simulink model "mtuner_process"  (Simulink 3.00)
libraries: mathlib x4, analoglib x3, genlib x2, execlib x1, modellib x1

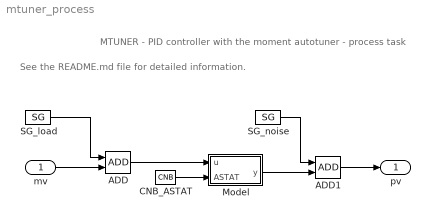
== system mtuner_process ==
  note: See the README.md file for detailed information.
  note: MTUNER - PID controller with the moment autotuner - process task
  mv : Inport  Port=1
  ADD : mathlib/ADD
  ADD1 : mathlib/ADD
  CNB_ASTAT : mathlib/CNB  YCN=off
  Model : Subsystem
      mask Type: REX sequence
  SG_load : genlib/SG  isig=1: SINE  amp=0  freq=0.01  phase=0  ifrunit=1: Hz  iphunit=1: DEGREE  offset=0
  SG_noise : genlib/SG  isig=4: RANDOM  amp=0  freq=0.01  phase=0  ifrunit=1: Hz  iphunit=1: DEGREE  offset=0
  pv : Outport  Port=1
  wires:
  ADD/1 -> Model/1(u)
  ADD1/1 -> pv/1
  CNB_ASTAT/1 -> Model/2(ASTAT)
  Model/1(y) -> ADD1/2
  SG_load/1 -> ADD/1
  SG_noise/1 -> ADD1/1
  mv/1 -> ADD/2

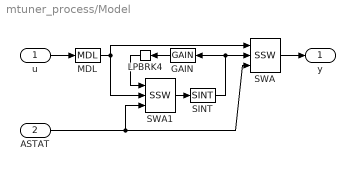
== system mtuner_process/Model ==
  u : Inport  Port=1
  ASTAT : Inport  Port=2
  GAIN : mathlib/GAIN  Orientation=left  k=-1
  LPBRK4 : execlib/LPBRK  Orientation=left
  MDL : modellib/MDL  k0=1  del=0  tau1=10  tau2=2  nmax=100
  SINT : analoglib/SINT  ti=1  y0=0  ymax=100  ymin=-100
  SWA : analoglib/SSW
  SWA1 : analoglib/SSW
  y : Outport  Port=1
  wires:
  ASTAT/1 -> SWA/3, SWA1/3
  GAIN/1 -> LPBRK4/1
  LPBRK4/1 -> SWA1/1
  MDL/1 -> SWA/1, SWA1/2
  SINT/1 -> GAIN/1, SWA/2
  SWA/1 -> y/1
  SWA1/1 -> SINT/1
  u/1 -> MDL/1
